simulink model "coupled_tanks_s_3C"  (R2015b)
settings: Solver=ode1  StartTime=0.0  StopTime=150  FixedStep=0.002  RelTol=1e-3
PostLoadFcn:
  | qc_set_target_type(getConfigSet(bdroot, 'QUARC Default Target Configuration'));
values from neighbouring files (symbols this model uses):
  A = [(-a1/A1)*sqrt(g/(2*L10)) 0;(a1/A2)*sqrt(g/(2*L10)) (-a2/A2)*sqrt(g/(2*L20)) ]    [seguidor_referencia_estados_estimado_3C.m]
  B = [Km/A1; 0]    [seguidor_referencia_estados_estimado_3C.m]
  C = [0 1]    [seguidor_referencia_estados_estimado_3C.m]
  K1 = K(1)    [seguidor_referencia_estados_estimado_3C.m]
  K2 = [K(2) K(3)]    [seguidor_referencia_estados_estimado_3C.m]
  L = real(qlA*inv(V)*[0;1])    [seguidor_referencia_estados_estimado_3C.m]
undefined symbols (not defined in the file or in its folder): HIL
libraries: simulink x6, quarc_library x3
settings Model: SimulationMode=external  ExtModeTrigDuration=30000  Creator=MLevis  LastModifiedBy=UFRN
settings SolverCC: PositivePriorityOrder=on
settings DataIOCC: SaveFormat=Array  SignalLoggingSaveFormat=ModelDataLogs
settings OptimizationCC: ExpressionDepthLimit=2147483647  InitFltsAndDblsToZero=on
settings DebuggingCC: SaveWithParameterizedLinksMsg=none  UnderspecifiedInitializationDetection=Classic  MergeDetectMultiDrivingBlocksExec=none  SolverPrmCheckMsg=warning  MultiTaskDSMMsg=warning  MultiTaskCondExecSysMsg=none  FcnCallInpInsideContextMsg=UseLocalSettings  StateNameClashWarn=warning
settings HardwareCC: ProdBitPerPointer=32  ProdLargestAtomicFloat=None  ProdIntDivRoundTo=Undefined  ProdEndianess=Unspecified  ProdWordSize=32  ProdHWDeviceType=32-bit Generic
settings RTWCC: SystemTargetFile=quarc_win64.tlc  TemplateMakefile=quarc_default_tmf  Description=QUARC Win64 Target
settings GRTTargetCC: ParMdlRefBuildCompliant=off  CompOptLevelCompliant=off  GeneratePreprocessorConditionals=Disable all  CombineOutputUpdateFcns=off  MatFileLogging=off  GRTInterface=on  UseToolchainInfoCompliant=off  ExtMode=on  ExtModeMexFile=quarc_comm
settings ConfigComp: CovModelRefEnable=Off

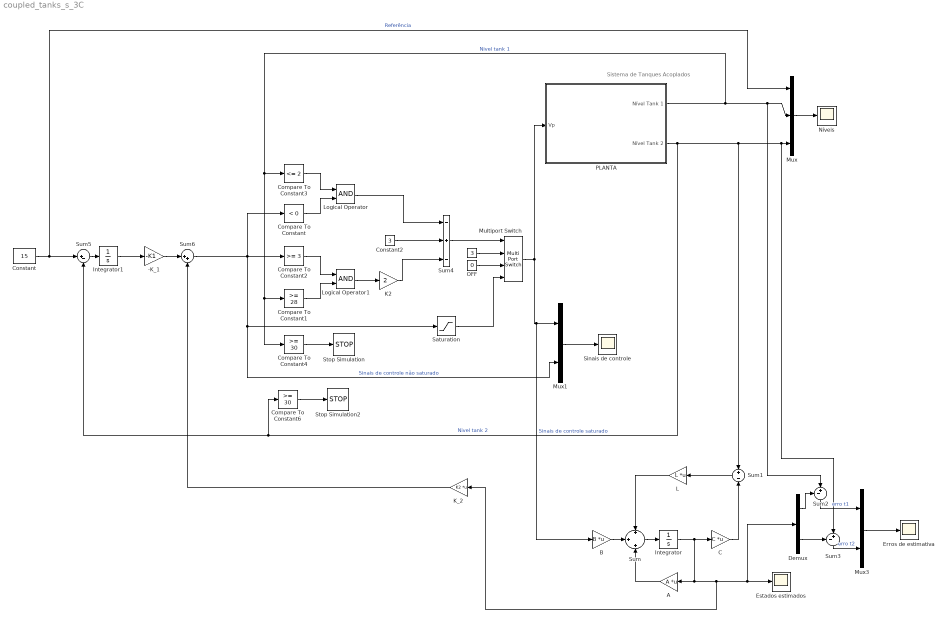
== system coupled_tanks_s_3C ==
  note: Sistema de Tanques Acoplados
  " " : Constant  Value=3
  "-K_1 " : Gain  Gain=-K1
  "A " : Gain  Gain=A  Multiplication=Matrix(K*u) (u vector)
  B : Gain  Gain=B  Multiplication=Matrix(K*u) (u vector)
  C : Gain  Gain=C  Multiplication=Matrix(K*u) (u vector)
  Compare To Constant : simulink/Logic and Bit Operations/Compare To Constant  relop=<  const=0  OutDataTypeStr=boolean
  Compare To Constant1 : simulink/Logic and Bit Operations/Compare To Constant  relop=>=  const=28  OutDataTypeStr=boolean
  Compare To Constant2 : simulink/Logic and Bit Operations/Compare To Constant  relop=>=  const=3  OutDataTypeStr=boolean
  Compare To Constant3 : simulink/Logic and Bit Operations/Compare To Constant  relop=<=  const=2  OutDataTypeStr=boolean
  Compare To Constant4 : simulink/Logic and Bit Operations/Compare To Constant  relop=>=  const=30  OutDataTypeStr=boolean
  Compare To Constant6 : simulink/Logic and Bit Operations/Compare To Constant  relop=>=  const=30  OutDataTypeStr=boolean
  Constant : Constant  Value=15
  Constant2 : Constant  Value=3
  Demux : Demux  Outputs=2
  Erros de estimativa : Scope
  Estados estimados : Scope
  Integrator : Integrator
  Integrator1 : Integrator
  K2 : Gain  Gain=2
  K_2 : Gain  Gain=K2  Multiplication=Matrix(K*u) (u vector)
  L : Gain  Gain=L  Multiplication=Matrix(K*u) (u vector)
  Logical Operator : Logic  AllPortsSameDT=off  OutDataTypeStr=boolean
  Logical Operator1 : Logic  AllPortsSameDT=off  OutDataTypeStr=boolean
  Multiport Switch : MultiPortSwitch
  Mux : Mux  Inputs=3
  Mux1 : Mux  Inputs=2
  Mux3 : Mux  Inputs=2
  Níveis : Scope
  OFF : Constant  Value=0
  PLANTA : Subsystem
  Saturation : Saturate  UpperLimit=4  LowerLimit=-4
  Sinais de controle : Scope
  Stop Simulation : Stop
  Stop Simulation2 : Stop
  Sum : Sum  Inputs=+|+|+
  Sum1 : Sum  Inputs=+-
  Sum2 : Sum  Inputs=-+|
  Sum3 : Sum  Inputs=-+|
  Sum4 : Sum  Inputs=-+-
  Sum5 : Sum  Inputs=|+-
  Sum6 : Sum  Inputs=|++
  wires:
  PLANTA/1(Nível Tank 1) -> Sum2/2, Mux/2, Compare To Constant3/1, Compare To Constant4/1, Compare To Constant1/1  "Nivel tank 1"
  Mux/1 -> Níveis/1
  PLANTA/2(Nível Tank 2) -> Sum1/1, Sum3/2, Mux/3, Sum5/2, Compare To Constant6/1  "Nivel tank 2"
  Mux1/1 -> Sinais de controle/1
  Constant/1 -> Mux/1, Sum5/1  "Referência"
  Compare To Constant3/1 -> Logical Operator/1
  Compare To Constant/1 -> Logical Operator/2
  Compare To Constant2/1 -> Logical Operator1/1
  Compare To Constant1/1 -> Logical Operator1/2
  Logical Operator/1 -> Sum4/1
  Logical Operator1/1 -> K2/1
  K2/1 -> Sum4/3
  Constant2/1 -> Sum4/2
  Compare To Constant4/1 -> Stop Simulation/1
  Sum4/1 -> Multiport Switch/1
  " "/1 -> Multiport Switch/2
  OFF/1 -> Multiport Switch/3
  Multiport Switch/1 -> B/1, Mux1/1, PLANTA/1(Vp)  "Sinais de controle saturado"
  Sum5/1 -> Integrator1/1
  Integrator1/1 -> "-K_1 "/1
  "-K_1 "/1 -> Sum6/1
  Sum6/1 -> Mux1/2, Saturation/1, Compare To Constant2/1, Compare To Constant/1  "Sinais de controle não saturado"
  Compare To Constant6/1 -> Stop Simulation2/1
  K_2/1 -> Sum6/2
  Saturation/1 -> Multiport Switch/4
  Mux3/1 -> Erros de estimativa/1
  B/1 -> Sum/2
  "A "/1 -> Sum/3
  L/1 -> Sum/1
  Sum/1 -> Integrator/1
  Integrator/1 -> K_2/1, Demux/1, Estados estimados/1, "A "/1, C/1
  Sum1/1 -> L/1
  C/1 -> Sum1/2
  Demux/1 -> Sum2/1
  Sum2/1 -> Mux3/1  "erro t1"
  Demux/2 -> Sum3/1
  Sum3/1 -> Mux3/2  "erro t2"

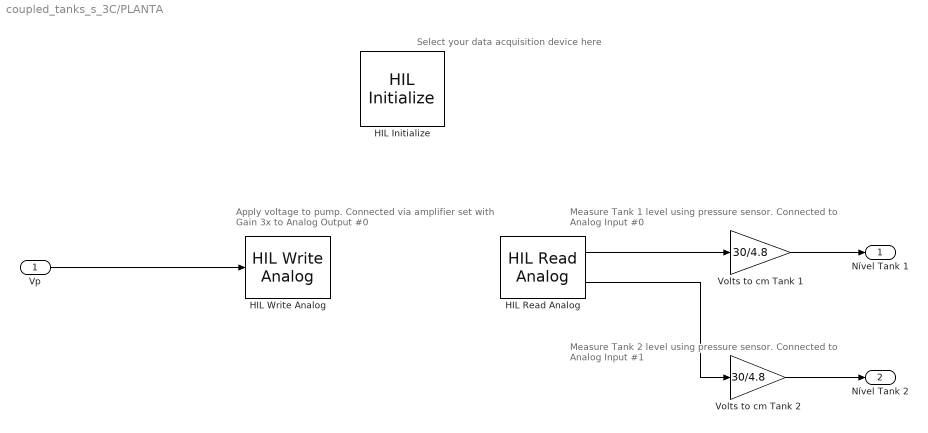
== system coupled_tanks_s_3C/PLANTA ==
  note: Select your data acquisition device here
  note: Apply voltage to pump.
      | Connected via amplifier set with Gain 3x
      | to  Analog Output #0
  note: Measure Tank 2 level using pressure sensor.
      | Connected to Analog Input #1
  note: Measure Tank 1 level using pressure sensor.
      | Connected to Analog Input #0
  Vp : Inport
  HIL Initialize : quarc_library/Data Acquisition/Generic/Configuration/HIL Initialize  object_name=HIL-1  board_type=q8_usb  board_number=0  board_options=update_rate=normal;decimation=1  exclusive=off  active=off  hardware_clocks=[0:2]  clock_modes=[]  initial_clock_frequencies=[]  set_clock_params_at_start=off  set_clock_params_at_switch_in=off  set_clock_frequencies_at_start=off  set_clock_frequencies_at_switch_in=off  analog_input_channels=[0:7]  analog_input_maximums=10  analog_input_minimums=-10  set_analog_input_params_at_start=on  set_analog_input_params_at_switch_in=off  analog_output_channels=[0:7]  analog_output_maximums=10  analog_output_minimums=-10  initial_analog_outputs=[0]  final_analog_outputs=[0]  watchdog_analog_outputs=0  set_analog_output_params_at_start=on  set_analog_output_params_at_switch_in=off  set_analog_outputs_at_start=on  set_analog_outputs_at_switch_in=off  set_analog_outputs_at_terminate=on  set_analog_outputs_at_switch_out=off  set_analog_outputs_on_watchdog=off  digital_input_channels=[]  digital_output_channels=[]  digital_output_configuration=[]  initial_digital_outputs=[1]  final_digital_outputs=[1]  watchdog_digital_outputs=[1]  set_digital_output_params_at_start=off  set_digital_output_params_at_switch_in=off  set_digital_outputs_at_start=on  set_digital_outputs_at_switch_in=off  set_digital_outputs_at_terminate=on  set_digital_outputs_at_switch_out=off  set_digital_outputs_on_watchdog=off  encoder_channels=[0:7]  quadrature=[4]  encoder_filter_frequency=[]  initial_encoder_counts=[0]  set_encoder_params_at_start=on  set_encoder_params_at_switch_in=off  set_encoder_counts_at_start=on  set_encoder_counts_at_switch_in=off  pwm_channels=[0:7]  pwm_modes=0  pwm_frequency=99.532799999999995e6/4095  pwm_configuration=[0]  pwm_alignment=[0]  pwm_polarity=[1]  pwm_leading_deadband=[0]  pwm_trailing_deadband=[0]  initial_pwm_outputs=[0]  final_pwm_outputs=[0]  watchdog_pwm_outputs=[0]  set_pwm_params_at_start=on  set_pwm_params_at_switch_in=off  set_pwm_outputs_at_start=on  set_pwm_outputs_at_switch_in=off  set_pwm_outputs_at_terminate=on  set_pwm_outputs_at_switch_out=off  set_pwm_outputs_on_watchdog=off  other_output_channels=[]  initial_other_outputs=[]  final_other_outputs=[]  watchdog_other_outputs=[]  set_other_outputs_at_start=off  set_other_outputs_at_switch_in=off  set_other_outputs_at_terminate=off  set_other_outputs_at_switch_out=off  set_other_outputs_on_watchdog=off
  HIL Read Analog : quarc_library/Data Acquisition/Generic/Immediate I//O/HIL Read Analog  object_name=HIL-1  channels=[0:1]  sample_time=qc_get_step_size  active=on  vector_output=off
  HIL Write Analog : quarc_library/Data Acquisition/Generic/Immediate I//O/HIL Write Analog  object_name=HIL-1  channels=0  sample_time=-1  active=off  vector_input=off
  "Volts to cm Tank 1 " : Gain  Gain=30/4.8
  Volts to cm Tank 2 : Gain  Gain=30/4.8
  Nível Tank 1 : Outport
  Nível Tank 2 : Outport  Port=2
  wires:
  HIL Read Analog/1 -> "Volts to cm Tank 1 "/1
  HIL Read Analog/2 -> Volts to cm Tank 2/1
  Vp/1 -> HIL Write Analog/1
  "Volts to cm Tank 1 "/1 -> Nível Tank 1/1
  Volts to cm Tank 2/1 -> Nível Tank 2/1
